simulink model "Batter_Modelling_step_discharge_2017A (1)"  (R2017a)
settings: Solver=VariableStepAuto  StartTime=0.0  StopTime=3600  RelTol=1e-3
libraries: simulink x2
settings Model: Creator=Darshan  LastModifiedBy=srajuvel

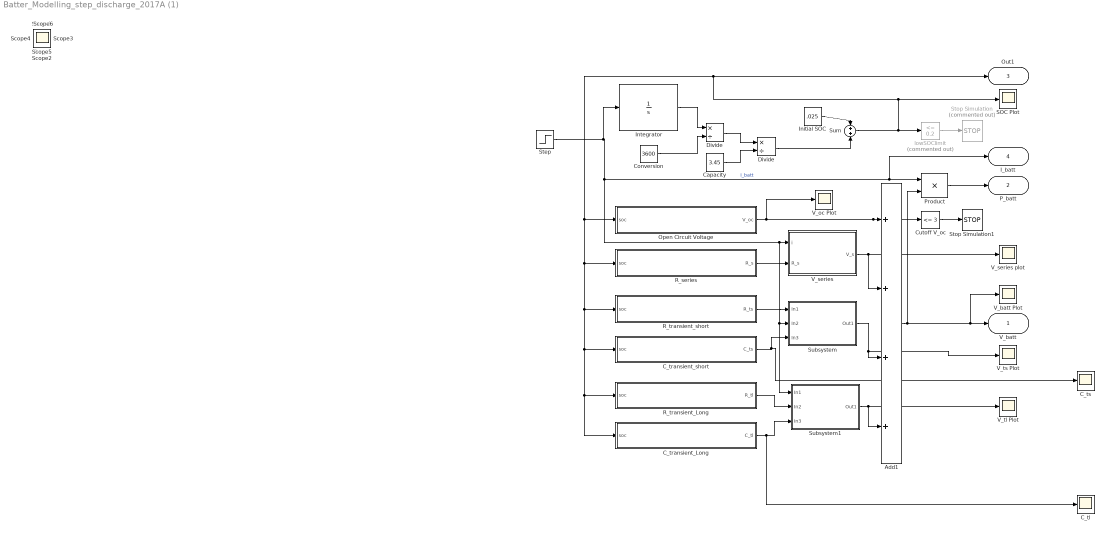
== system Batter_Modelling_step_discharge_2017A (1) ==
  Add1 : Sum  Inputs=++++
  C_tl : Scope
  C_transient_Long : MATLAB Function  TreatAsAtomicUnit=on
  C_transient_short : MATLAB Function  TreatAsAtomicUnit=on
  C_ts : Scope
  "Capacity " : Constant  Value=3.45  SampleTime=1
  Conversion : Constant  Value=3600  SampleTime=1
  Cutoff V_oc : simulink/Logic and Bit Operations/Compare To Constant  relop=<=  const=3  OutDataTypeStr=boolean
  Divide : Product  Inputs=*/
  "Divide " : Product  Inputs=*/
  Initial SOC : Constant  Value=.025  SampleTime=1
  Integrator : Integrator  InitialCondition=1
  Open Circuit Voltage : MATLAB Function  TreatAsAtomicUnit=on
  Product : Product
  R_series : MATLAB Function  TreatAsAtomicUnit=on
  R_transient_Long : MATLAB Function  TreatAsAtomicUnit=on
  R_transient_short : MATLAB Function  TreatAsAtomicUnit=on
  "SOC Plot " : Scope
  Step : Step  Time=3600  Before=3.45  After=0  SampleTime=0.01
  Stop Simulation : Stop  Commented=on
  Stop Simulation1 : Stop
  Subsystem : Subsystem
  Subsystem1 : Subsystem
  Sum : Sum
  "V_batt Plot " : Scope
  "V_oc Plot " : Scope
  V_series : MATLAB Function  TreatAsAtomicUnit=on
  "V_series plot " : Scope
  V_tl Plot : Scope
  "V_ts Plot " : Scope
  lowSOClimit : simulink/Logic and Bit Operations/Compare To Constant  Commented=on  relop=<=  const=0.2  OutDataTypeStr=boolean
  V_batt : Outport
  P_batt : Outport  Port=2
  Out1 : Outport  Port=3
  I_batt : Outport  Port=4
  Scope{,1..6} (7 alike) : Scope
  wires:
  R_series/1(R_s) -> V_series/2(R_s)
  Subsystem1/1(Out1) -> Add1/4, V_tl Plot/1
  V_series/1(V_s) -> "V_series plot "/1, Add1/2
  Product/1 -> P_batt/1
  Step/1 -> Subsystem1/1(In1), Subsystem/2(In2), V_series/1(i), I_batt/1, Product/1, Integrator/1  "I_batt"
  C_transient_Long/1(C_tl) -> C_tl/1, Subsystem1/3(In3)
  R_transient_Long/1(R_tl) -> Subsystem1/2(In2)
  Open Circuit Voltage/1(V_oc) -> "V_oc Plot "/1, Add1/1, Cutoff V_oc/1
  C_transient_short/1(C_ts) -> C_ts/1, Subsystem/3(In3)
  Sum/1 -> lowSOClimit/1, C_transient_Long/1(soc), R_transient_Long/1(soc), C_transient_short/1(soc), R_transient_short/1(soc), R_series/1(soc), Open Circuit Voltage/1(soc), Out1/1, "SOC Plot "/1
  lowSOClimit/1 -> Stop Simulation/1
  Conversion/1 -> "Divide "/2
  "Capacity "/1 -> Divide/2
  Initial SOC/1 -> Sum/1
  Integrator/1 -> "Divide "/1
  "Divide "/1 -> Divide/1
  Cutoff V_oc/1 -> Stop Simulation1/1
  Add1/1 -> Product/2, "V_batt Plot "/1, V_batt/1
  R_transient_short/1(R_ts) -> Subsystem/1(In1)
  Subsystem/1(Out1) -> "V_ts Plot "/1, Add1/3
  Divide/1 -> Sum/2

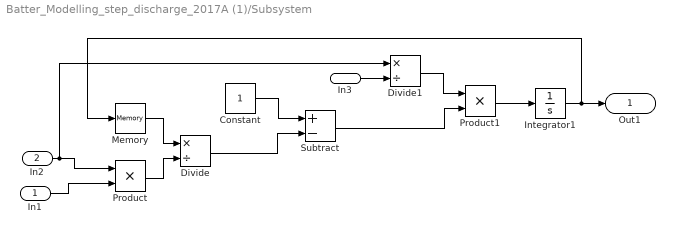
== system Batter_Modelling_step_discharge_2017A (1)/Subsystem ==
  In1 : Inport
  In2 : Inport  Port=2
  In3 : Inport  Port=3
  Constant : Constant
  Divide : Product  Inputs=*/
  Divide1 : Product  Inputs=*/
  Integrator1 : Integrator
  Memory : Memory
  Product : Product
  Product1 : Product
  Subtract : Sum  Inputs=+-
  Out1 : Outport
  wires:
  In1/1 -> Product/2
  In2/1 -> Divide1/1, Product/1
  In3/1 -> Divide1/2
  Product/1 -> Divide/2
  Constant/1 -> Subtract/1
  Divide/1 -> Subtract/2
  Divide1/1 -> Product1/1
  Subtract/1 -> Product1/2
  Memory/1 -> Divide/1
  Product1/1 -> Integrator1/1
  Integrator1/1 -> Memory/1, Out1/1

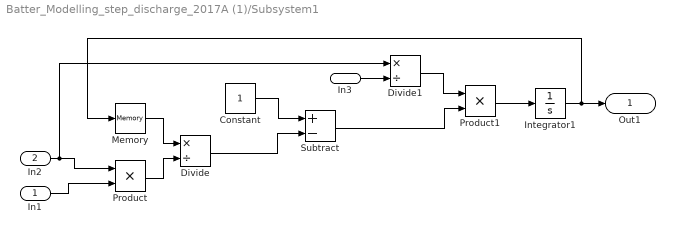
== system Batter_Modelling_step_discharge_2017A (1)/Subsystem1 ==
  In1 : Inport
  In2 : Inport  Port=2
  In3 : Inport  Port=3
  Constant : Constant
  Divide : Product  Inputs=*/
  Divide1 : Product  Inputs=*/
  Integrator1 : Integrator
  Memory : Memory
  Product : Product
  Product1 : Product
  Subtract : Sum  Inputs=+-
  Out1 : Outport
  wires:
  In1/1 -> Product/2
  In2/1 -> Divide1/1, Product/1
  In3/1 -> Divide1/2
  Product/1 -> Divide/2
  Constant/1 -> Subtract/1
  Divide/1 -> Subtract/2
  Divide1/1 -> Product1/1
  Subtract/1 -> Product1/2
  Memory/1 -> Divide/1
  Product1/1 -> Integrator1/1
  Integrator1/1 -> Memory/1, Out1/1

== matlab function Batter_Modelling_step_discharge_2017A (1)/R_series ==
  data: soc input; R_s output
function R_s = fcn(soc)

R_s = 0.1562*exp(-24.37*soc)+0.07446;

== matlab function Batter_Modelling_step_discharge_2017A (1)/Open Circuit Voltage ==
  data: soc input; V_oc output
function V_oc = fcn(soc)
%#codegen

%syms soc
V_oc = -1.031*exp(-35*soc) + 3.685 + 0.2156*soc - 0.1178*soc^2 + 0.3201*soc^3;
%soc = 0.0:0.01:1.0;
%SOC = meshgrid(soc);
%plot(SOC(1,:),subs(V_oc,soc(1,:)));

== matlab function Batter_Modelling_step_discharge_2017A (1)/R_transient_short ==
  data: soc input; R_ts output
function R_ts = fcn(soc)

R_ts = 0.3208*exp(-29.14*soc)+0.04669;

== matlab function Batter_Modelling_step_discharge_2017A (1)/C_transient_short ==
  data: soc input; C_ts output
function C_ts = fcn(soc)

C_ts = -752.9*exp(-13.51*soc)+703.6;

== matlab function Batter_Modelling_step_discharge_2017A (1)/R_transient_Long ==
  data: soc input; R_tl output
function R_tl = fcn(soc)

R_tl = 6.603*exp(-155.2*soc)+0.04984;

== matlab function Batter_Modelling_step_discharge_2017A (1)/C_transient_Long ==
  data: soc input; C_tl output
function C_tl = fcn(soc)

C_tl = -6065*exp(-27.12*soc)+4475;

== matlab function Batter_Modelling_step_discharge_2017A (1)/V_series ==
  data: i input; V_s output; R_s input
function V_s = fcn(i,R_s)

V_s = i*R_s;
